simulink model "DC_simulink"  (R2024b)
settings: Solver=VariableStepAuto  StartTime=0.0  StopTime=10.0  RelTol=1e-3
values from neighbouring files (symbols this model uses):
  b = 0.0012    [DC.m]    (also in DC_parametros.m)
  J = 0.001    [DC.m]    (also in DC_parametros.m)
  Ke = 0.01    [DC.m]    (also in DC_parametros.m)
  Kt = 0.01    [DC.m]    (also in DC_parametros.m)
  La = 0.023    [DC.m]    (also in DC_parametros.m)
  Ra = 2    [DC.m]    (also in DC_parametros.m)
settings Model: Creator=Aguirre

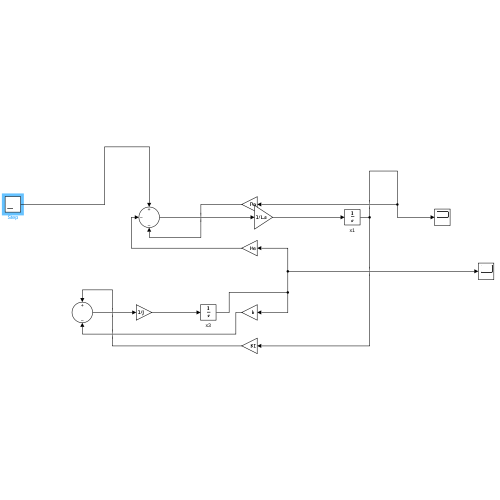
[thumbnail: Simulink's stored preview of the top-level diagram]
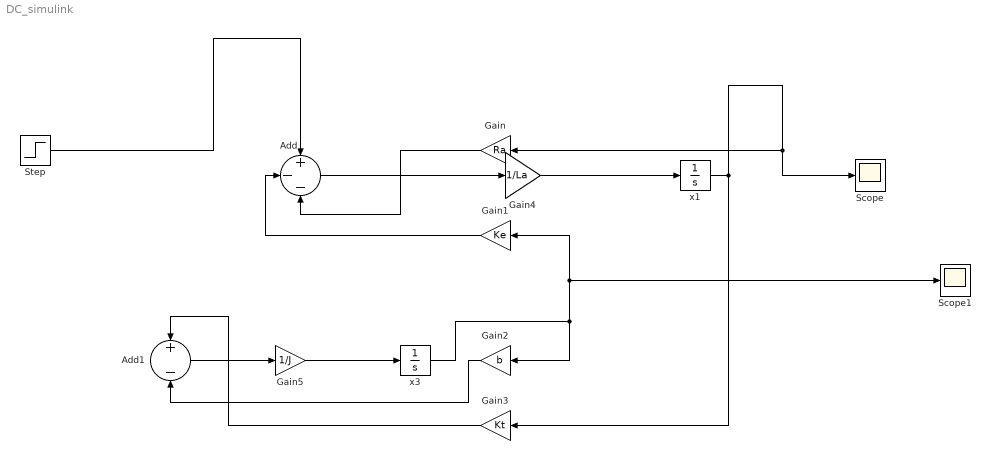
== system DC_simulink ==
  Add : Sum  Inputs=+--
  Add1 : Sum  Inputs=+-
  Gain : Gain  Gain=Ra
  Gain1 : Gain  Gain=Ke
  Gain2 : Gain  Gain=b
  Gain3 : Gain  Gain=Kt
  Gain4 : Gain  Gain=1/La
  Gain5 : Gain  Gain=1/J
  Scope : Scope
  Scope1 : Scope
  Step : Step  Time=0  After=10  SampleTime=0
  x1 : Integrator
  x3 : Integrator
  wires:
  Gain1/1 -> Add/2
  Gain3/1 -> Add1/1
  Gain2/1 -> Add1/2
  Gain5/1 -> x3/1
  Add1/1 -> Gain5/1
  x1/1 -> Scope/1, Gain/1, Gain3/1
  Gain/1 -> Add/3
  x3/1 -> Gain1/1, Scope1/1, Gain2/1
  Gain4/1 -> x1/1
  Add/1 -> Gain4/1
  Step/1 -> Add/1
